simulink model "control_pid"  (R2015a)
settings: Solver=ode45  StartTime=0.0  StopTime=50  RelTol=1e-3
PreLoadFcn:
  | parameters
undefined symbols (not defined in the file or in its folder): Ch, D, Ke, Kh, L, M1, R
settings Model: Creator=dell  LastModifiedBy=dell

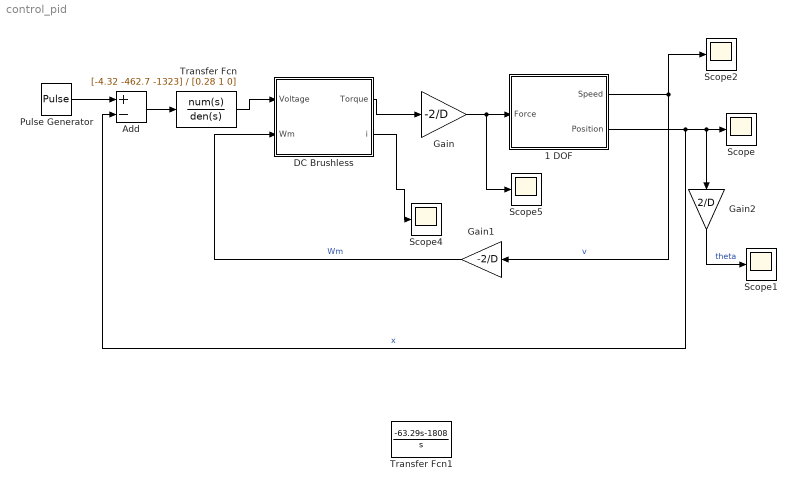
== system control_pid ==
  "1 DOF " : Subsystem
  Add : Sum  Inputs=+-
  DC Brushless : Subsystem
  Gain : Gain  Gain=-2/D
  Gain1 : Gain  Gain=-2/D
  Gain2 : Gain  Gain=2/D
  Pulse Generator : DiscretePulseGenerator  PulseType=Time based  Period=10  PulseWidth=50
  Scope{,1..2,4..5} (5 alike) : Scope
      Scope settings: TimeRange=20  YMin=-6.5e+295  YMax=5e+295
      Scope1 settings: TimeRange=20  YMin=0  YMax=0.0015
      Scope2 settings: TimeRange=20  YMin=1.5e-06  YMax=5.75e-06  SaveName=ScopeData3
      Scope4 settings: TimeRange=20  YMin=1.5e-06  YMax=5.75e-06  SaveName=ScopeData6
      Scope5 settings: TimeRange=23.33  YMin=-4  YMax=4  SaveName=ScopeData7
  Transfer Fcn : TransferFcn  Numerator=[-4.32 -462.7 -1323]  Denominator=[0.28 1 0]
  Transfer Fcn1 : TransferFcn  Numerator=[-63.29 -1808]  Denominator=[1 0]
  wires:
  DC Brushless/1("Torque ") -> Gain/1
  Gain/1 -> Scope5/1, "1 DOF "/1(Force)
  Gain1/1 -> DC Brushless/2(Wm)  "Wm"
  "1 DOF "/1("Speed ") -> Gain1/1, Scope2/1  "v"
  "1 DOF "/2("Position ") -> Add/2, Gain2/1, Scope/1  "x"
  Gain2/1 -> Scope1/1  "theta"
  DC Brushless/2("i ") -> Scope4/1
  Pulse Generator/1 -> Add/1
  Add/1 -> Transfer Fcn/1
  Transfer Fcn/1 -> DC Brushless/1("Voltage ")

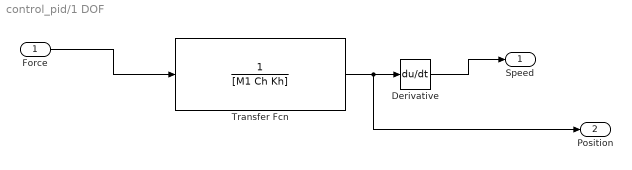
== system control_pid/1 DOF  ==
  Force : Inport
  Derivative : Derivative
  Transfer Fcn : TransferFcn  Denominator=[M1 Ch Kh]
  "Speed " : Outport
  "Position " : Outport  Port=2
  wires:
  Force/1 -> Transfer Fcn/1
  Transfer Fcn/1 -> "Position "/1, Derivative/1
  Derivative/1 -> "Speed "/1

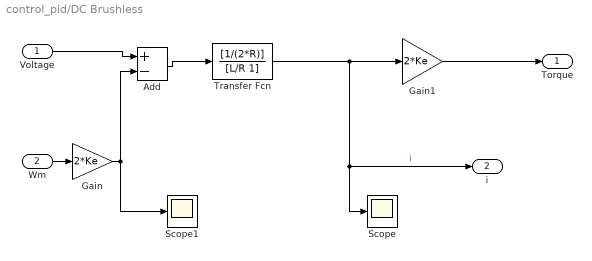
== system control_pid/DC Brushless ==
  "Voltage " : Inport
  Wm : Inport  Port=2
  Add : Sum  Inputs=+-
  Gain : Gain  Gain=2*Ke
  Gain1 : Gain  Gain=2*Ke
  Scope : Scope
      settings: YMin=-0.075  YMax=0.125  SaveName=ScopeData2
  Scope1 : Scope
      settings: YMin=-0.35  YMax=0.35  SaveName=ScopeData4
  Transfer Fcn : TransferFcn  Numerator=[1/(2*R)]  Denominator=[L/R 1]
  "Torque " : Outport
  "i " : Outport  Port=2
  wires:
  Gain1/1 -> "Torque "/1
  Transfer Fcn/1 -> "i "/1, Scope/1, Gain1/1  "i"
  Add/1 -> Transfer Fcn/1
  "Voltage "/1 -> Add/1
  Wm/1 -> Gain/1
  Gain/1 -> Scope1/1, Add/2
